simulink model "dspmrf_nlp"  (Simulink 5.0)
settings: Solver=FixedStepDiscrete  SolverMode=SingleTasking  StartTime=0.0  StopTime=inf  RelTol=1e-3  AbsTol=1e-6
PreLoadFcn:
  | load dspmrf_coeffs
libraries: dspmlti3 x4, dspsrcs4 x1, dspmrf_lib x1
settings Model: Creator=don  LastModifiedBy=schim  ExtModeTrigMode=oneshot  ExtModeArmWhenConnect=off  SaveTime=off  SaveOutput=off  LimitDataPoints=off  IntegerOverflowMsg=none  BlockReductionOpt=off  BooleanDataType=off  RTWOptions=-aRollThreshold=2

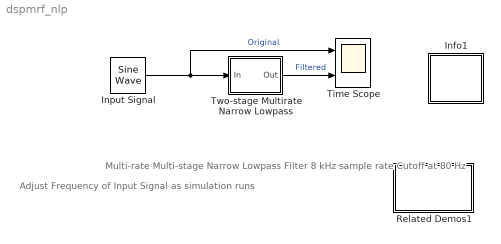
== system dspmrf_nlp ==
  note: Multi-rate Multi-stage
      | Narrow Lowpass Filter
      |
      | 8 kHz sample rate
      | Cutoff at 80 Hz
  note: Adjust Frequency
      | of Input Signal
      | as simulation runs
  Info1 : Subsystem
      mask Display: disp('Info')
  Input Signal : dspsrcs4/Sine Wave  Amplitude=1  Frequency=40  Phase=0  SampleMode=Discrete  OutComplex=Real  CompMethod=Trigonometric fcn  TableSize=Speed  SampleTime=1/8000  SamplesPerFrame=1  dataType=double  wordLen=16  udDataType=sfix(16)  fracBitsMode=Best precision  numFracBits=14  ResetState=Restart at time zero
  Related Demos1 : Subsystem
      settings: OpenFcn=dspmrf_menu
      mask Display: disp('Other\nMultirate Filter\nDemos')
  Time Scope : Scope  NumInputPorts=2
      settings: TimeRange=1.5  YMin=-1.5~-1.5  YMax=1.5~1.5  DataFormat=Structure
  Two-stage Multirate Narrow Lowpass : Subsystem
  wires:
  Input Signal/1 -> Time Scope/1, Two-stage Multirate Narrow Lowpass/1(In)  "Original"
  Two-stage Multirate Narrow Lowpass/1(Out) -> Time Scope/2  "Filtered"

== system dspmrf_nlp/Info1 ==
  note: Thi s example demonstrates the use of multiple stages of decimation to
      | achieve filtering with very short bandwidths and low computational loads.
      |
      | In this example, assume that the input signal has a maximum bandwidth
      | of 4 kHz, and is sampled at 8 kHz.  We wish to isolate signals located in the
      | lower 75 Hz region of the spectrum with a transition band from 75 to 80
      | The maximum passband ripple must be 0.01 and stopband ripple 1E-4.
      |
      | To achieve this specification with a single filter and no decimation, an
      | equiripple filter of length  "remezord([75 80], [1 0], [1E-2 1E-4], 8000)"
      | or 5022 is required, a very long filter with high computational load.
  note: Multistage Multirate FIR Filtering
  note: Alternatively, note that a signal with maximum bandwidth 80 Hz
      | is highly oversampled at 8 kHz; at a minimal sample rate of 2*80 Hz, a
      | decimation factor of 8000/160 = 50 could be employed.  We'll use
      | a total decimation factor of 48.
      |
      | Choosing to decimate the signal in two stages (D1=12 and D2=4),
      | the first stage must employ a lowpass filter with normalized cutoff
      | of 1/12.  The required filter length is found from remezord:
      |  "remezord([1/12-.01 1/12],[1 0], [0.5E-2 1E-4], 2)"
      | or 675, where we halved the allowed passband ripple since
      | a second filter stage must be employed.
      |
      | The second stage filter length requirement
      | is "remezord([75 80],[1 0],[0.5E-2 1E-4], 8000/12)" or 450.
      |
      | Total number of filter taps is 1127.  The computation rate has also
      | been reduced dramatically, since the first stage filter runs at 1/12 the
      | rate of the input signal, and the second stage filter runs at 1/48 of this rate.

== system dspmrf_nlp/Related Demos1 ==

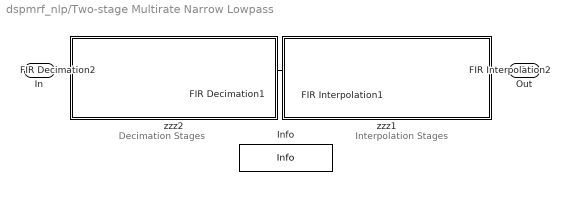
== system dspmrf_nlp/Two-stage Multirate Narrow Lowpass ==
  note: Interpolation Stages
  note: Decimation Stages
  In : Inport
  FIR Decimation1 : dspmlti3/FIR Decimation  h=mrf_firdn2  D=4  framing=Maintain input frame size  outputBufInitCond=0
  FIR Decimation2 : dspmlti3/FIR Decimation  h=mrf_firdn1  D=12  framing=Maintain input frame size  outputBufInitCond=0
  FIR Interpolation1 : dspmlti3/FIR Interpolation  h=mrf_upfir2  L=4  framing=Maintain input frame size  outputBufInitCond=0
  FIR Interpolation2 : dspmlti3/FIR Interpolation  h=mrf_upfir1  L=12  framing=Maintain input frame size  outputBufInitCond=0
  Info : dspmrf_lib/Info
  zzz1 : Subsystem
      settings: OpenFcn=dspmsmrff;
      mask Display: disp('')
  zzz2 : Subsystem
      settings: OpenFcn=dspmsmrff;
      mask Display: disp('')
  Out : Outport
  wires:
  FIR Interpolation2/1 -> Out/1
  FIR Interpolation1/1 -> FIR Interpolation2/1
  FIR Decimation1/1 -> FIR Interpolation1/1
  FIR Decimation2/1 -> FIR Decimation1/1
  In/1 -> FIR Decimation2/1

== system dspmrf_nlp/Two-stage Multirate Narrow Lowpass/zzz1 ==

== system dspmrf_nlp/Two-stage Multirate Narrow Lowpass/zzz2 ==
